simulink model "radiator_model_DOE"  (R2023b)
settings: Solver=FixedStepAuto  StartTime=0.0  StopTime=1200  FixedStep=0.244  RelTol=1e-3
InitFcn:
  | EngHeatRe2EngColnt=2150;
  | ColntFlw=0.2;
  | ColntHeatCp=4200;
  | EngColntMss=5.5;
  | RadColntMss=2.56;
  | RadArea=0.93;
  | AirTemp=13;
  | RadOnFanHgain=9.75;
  | RadH=8;
  | FanOnTemp=91;
  | FanOffTemp=85;
  | TrmstTemp=77.3;
  | InitEngColntOutTemp=55.5;
  | InitRadColntOutTemp=60;
settings Model: Creator=m.sorkhi  LastModifiedBy=m.sorkhi
settings SolverCC: ZeroCrossAlgorithm=Adaptive
settings DebuggingCC: IgnoredZcDiagnostic=none

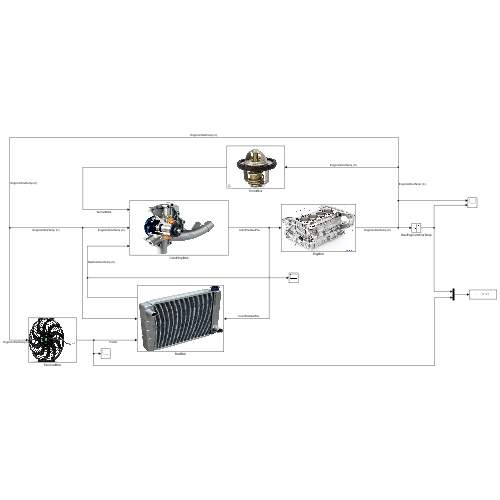
[thumbnail: Simulink's stored preview of the top-level diagram]
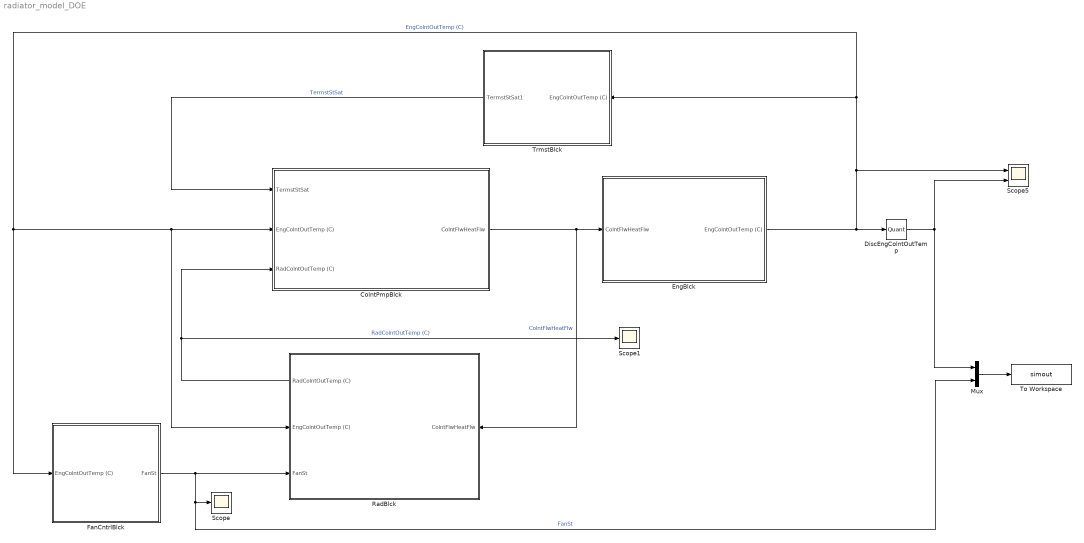
== system radiator_model_DOE ==
  ColntPmpBlck : Subsystem
      mask Display: image('wasserpumpe.jpg');
  DiscEngColntOutTemp : Quantizer  QuantizationInterval=0.75
  EngBlck : Subsystem
      mask Display: image('ICE_engine_block_details.jpg');
  FanCntrlBlck : Subsystem
      mask Display: image('71LbS5WTJxL._AC_UF1000,1000_QL80_.jpg');
  Mux : Mux  Inputs=2
  RadBlck : Subsystem
      settings: PortSchema="{\"entries\":[{\"content\":{\"sides\":[{\"content\":{\"connectorIds\":[\"Out1\",\"In1\",\"In2\"]},\"type\":\"ConnectorPlacement.EquallySpacedRectSide\",\"uuid\":\"5da9f111-79ac-4398-b2ca-ad7113d95e2a\"},{\"content\":{\"connectorIds\":[\"In3\"],\"side\":\"RIGHT\"},\"type\":\"ConnectorPlacement.EquallySpacedRectSide\",\"uuid\":\"beb3da66-0353-45dc-92dd-83812cc99847\"},{\"content\":{\"side\":\"TOP\"},\"type\":\"ConnectorPlacement.EquallySpacedRectSide\",\"uuid\":\"c3de1bb5-6f3a-4f20-91db-640cd95e3994\"}]},\"type\":\"ConnectorPlacement.EquallySpacedConnector\",\"uuid\":\"87d09cf3-4774-453a-a522-35e848abd666\"}],\"packageUris\":[\"http://schema.mathworks.com/mf0/Connector/R2020b\"],\"version\":\"1.0\"}"
      mask Display: image('Automobile_radiator.jpg');
  Scope : Scope
  Scope1 : Scope
  Scope5 : Scope  NumInputPorts=2
  To Workspace : ToWorkspace  VariableName=simout  SaveFormat=Timeseries  SampleTime=-1
  TrmstBlck : Subsystem
      settings: PortSchema="{\"entries\":[{\"content\":{\"sides\":[{\"content\":{\"connectorIds\":[\"Out1\"]},\"type\":\"ConnectorPlacement.EquallySpacedRectSide\",\"uuid\":\"06f11dda-685b-413c-afa7-1258c3976e74\"},{\"content\":{\"connectorIds\":[\"In1\"],\"side\":\"RIGHT\"},\"type\":\"ConnectorPlacement.EquallySpacedRectSide\",\"uuid\":\"2745f48e-69b2-4d48-9193-e2e306ca83ef\"},{\"content\":{\"side\":\"TOP\"},\"type\":\"ConnectorPlacement.EquallySpacedRectSide\",\"uuid\":\"b89a6614-c438-49fa-af5b-58ae8dde8402\"}]},\"type\":\"ConnectorPlacement.EquallySpacedConnector\",\"uuid\":\"ed9858cb-f051-4637-aafc-3b577e7d11cc\"}],\"packageUris\":[\"http://schema.mathworks.com/mf0/Connector/R2020b\"],\"version\":\"1.0\"}"
      mask DialogControl Control1 Prompt: (Add text here)
      mask Display: image('thermostat-a-cooling-system-spare-parts-for-cars-PLFZKVV-min.jpg');
  wires:
  DiscEngColntOutTemp/1 -> Scope5/2, Mux/1
  EngBlck/1(EngColntOutTemp (C)) -> TrmstBlck/1(EngColntOutTemp (C)), ColntPmpBlck/2(EngColntOutTemp (C)), RadBlck/1(EngColntOutTemp (C)), FanCntrlBlck/1(EngColntOutTemp (C)), Scope5/1, DiscEngColntOutTemp/1  "EngColntOutTemp (C)"
  ColntPmpBlck/1(ColntFlwHeatFlw) -> RadBlck/3(ColntFlwHeatFlw), EngBlck/1(ColntFlwHeatFlw)  "ColntFlwHeatFlw"
  RadBlck/1(RadColntOutTemp (C)) -> Scope1/1, ColntPmpBlck/3(RadColntOutTemp (C))  "RadColntOutTemp (C)"
  TrmstBlck/1(TermstStSat1) -> ColntPmpBlck/1(TermstStSat)  "TermstStSat"
  FanCntrlBlck/1(FanSt) -> Mux/2, Scope/1, RadBlck/2(FanSt)  "FanSt"
  Mux/1 -> To Workspace/1

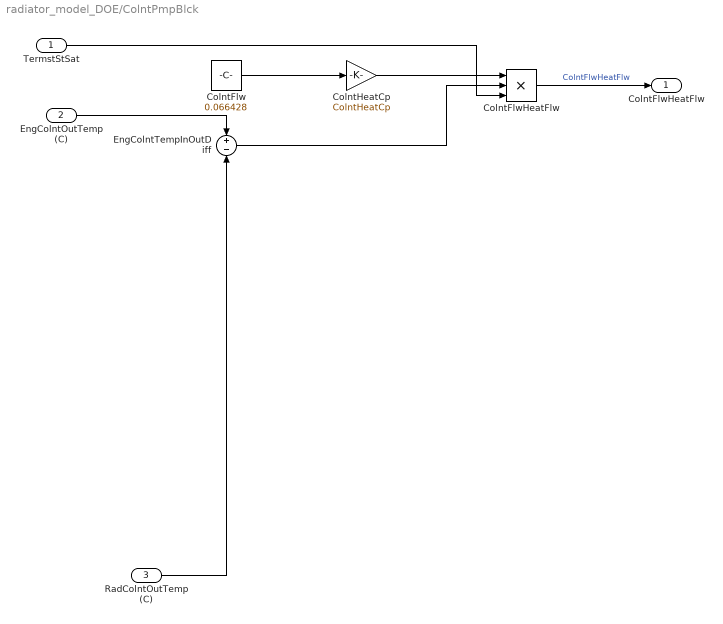
== system radiator_model_DOE/ColntPmpBlck ==
  TermstStSat : Inport
  EngColntOutTemp (C) : Inport  Port=2
  RadColntOutTemp (C) : Inport  Port=3
  ColntFlw : Constant  Value=0.066428
  "ColntFlwHeatFlw " : Product  Inputs=3
  ColntHeatCp : Gain  Gain=ColntHeatCp
  EngColntTempInOutDiff : Sum  Inputs=+-
  ColntFlwHeatFlw : Outport
  wires:
  "ColntFlwHeatFlw "/1 -> ColntFlwHeatFlw/1  "ColntFlwHeatFlw"
  ColntFlw/1 -> ColntHeatCp/1
  EngColntOutTemp (C)/1 -> EngColntTempInOutDiff/1
  ColntHeatCp/1 -> "ColntFlwHeatFlw "/1
  EngColntTempInOutDiff/1 -> "ColntFlwHeatFlw "/2
  TermstStSat/1 -> "ColntFlwHeatFlw "/3
  RadColntOutTemp (C)/1 -> EngColntTempInOutDiff/2

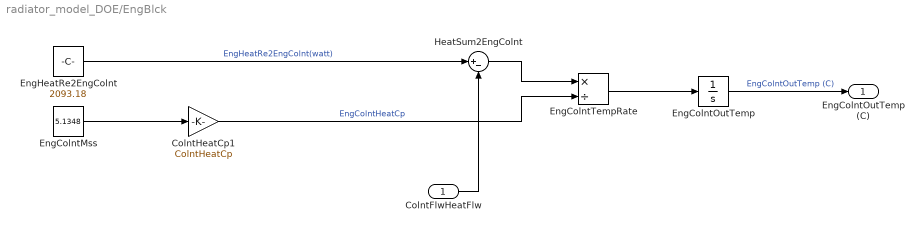
== system radiator_model_DOE/EngBlck ==
  ColntFlwHeatFlw : Inport
  ColntHeatCp1 : Gain  Gain=ColntHeatCp
  EngColntMss : Constant  Value=5.1348
  EngColntOutTemp : Integrator  InitialCondition=InitEngColntOutTemp
  EngColntTempRate : Product  Inputs=*/
  EngHeatRe2EngColnt : Constant  Value=2093.18
  HeatSum2EngColnt : Sum  Inputs=|+-
  EngColntOutTemp (C) : Outport
  wires:
  ColntHeatCp1/1 -> EngColntTempRate/2  "EngColntHeatCp"
  EngColntMss/1 -> ColntHeatCp1/1
  EngColntTempRate/1 -> EngColntOutTemp/1
  ColntFlwHeatFlw/1 -> HeatSum2EngColnt/2
  HeatSum2EngColnt/1 -> EngColntTempRate/1
  EngColntOutTemp/1 -> EngColntOutTemp (C)/1  "EngColntOutTemp (C)"
  EngHeatRe2EngColnt/1 -> HeatSum2EngColnt/1  "EngHeatRe2EngColnt(watt)"

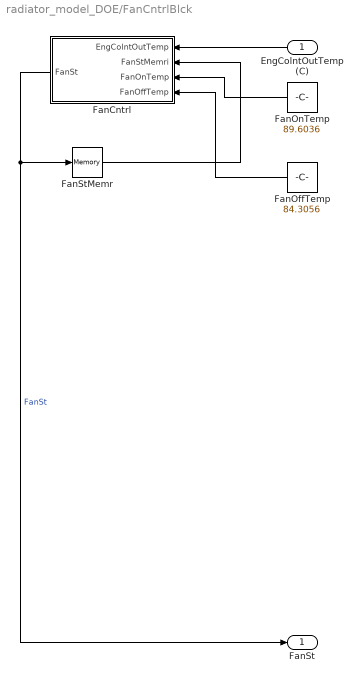
== system radiator_model_DOE/FanCntrlBlck ==
  EngColntOutTemp (C) : Inport
  FanCntrl : MATLAB Function  TreatAsAtomicUnit=on
  FanOffTemp : Constant  Value=84.3056
  FanOnTemp : Constant  Value=89.6036
  "FanStMemr " : Memory
  FanSt : Outport
  wires:
  FanCntrl/1(FanSt) -> FanSt/1, "FanStMemr "/1  "FanSt"
  "FanStMemr "/1 -> FanCntrl/2(FanStMemri)
  EngColntOutTemp (C)/1 -> FanCntrl/1(EngColntOutTemp)
  FanOffTemp/1 -> FanCntrl/4(FanOffTemp)
  FanOnTemp/1 -> FanCntrl/3(FanOnTemp)

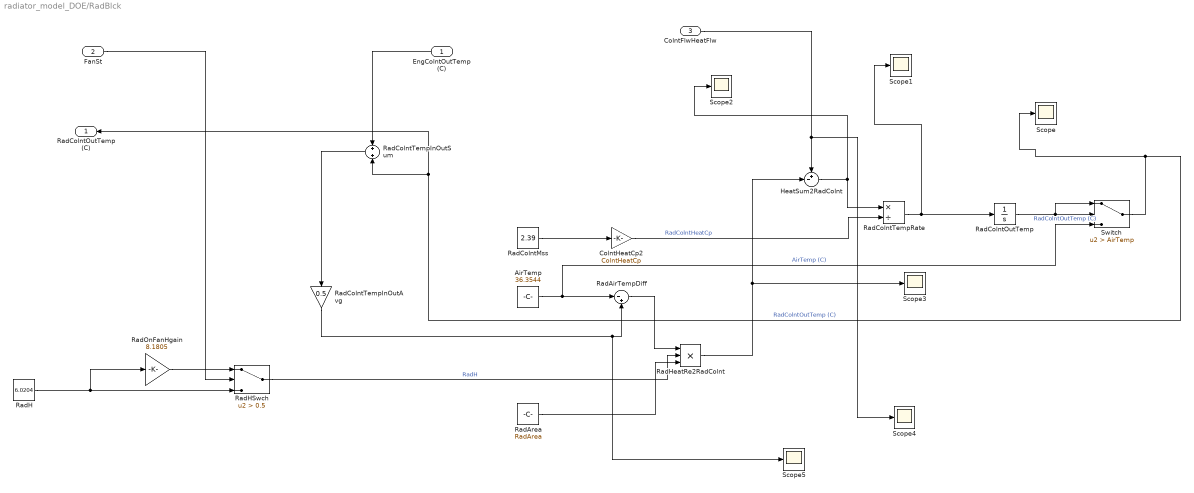
== system radiator_model_DOE/RadBlck ==
  EngColntOutTemp (C) : Inport
  FanSt : Inport  Port=2
  ColntFlwHeatFlw : Inport  Port=3
  AirTemp : Constant  Value=36.3544
  ColntHeatCp2 : Gain  Gain=ColntHeatCp
  HeatSum2RadColnt : Sum  Inputs=+-|
  RadAirTempDiff : Sum  Inputs=|-+
  RadArea : Constant  Value=RadArea
  RadColntMss : Constant  Value=2.39
  RadColntOutTemp : Integrator  InitialCondition=InitRadColntOutTemp
  RadColntTempInOutAvg : Gain  Gain=0.5
  RadColntTempInOutSum : Sum  Inputs=+|+
  RadColntTempRate : Product  Inputs=*/
  RadH : Constant  Value=6.0204
  RadHSwch : Switch  Criteria=u2 > Threshold  Threshold=0.5  SaturateOnIntegerOverflow=off  InputSameDT=off
  RadHeatRe2RadColnt : Product  Inputs=3
  RadOnFanHgain : Gain  Gain=8.1805
  Scope{,1..5} (6 alike) : Scope
  Switch : Switch  Criteria=u2 > Threshold  Threshold=AirTemp  SaturateOnIntegerOverflow=off  InputSameDT=off
  RadColntOutTemp (C) : Outport
  wires:
  RadColntTempInOutAvg/1 -> Scope5/1, RadAirTempDiff/2
  AirTemp/1 -> Switch/3, RadAirTempDiff/1  "AirTemp (C)"
  RadAirTempDiff/1 -> RadHeatRe2RadColnt/1
  RadColntMss/1 -> ColntHeatCp2/1
  Switch/1 -> Scope/1, RadColntOutTemp (C)/1, RadColntTempInOutSum/2  "RadColntOutTemp (C)"
  RadHeatRe2RadColnt/1 -> HeatSum2RadColnt/2, Scope3/1
  HeatSum2RadColnt/1 -> RadColntTempRate/1, Scope2/1
  RadHSwch/1 -> RadHeatRe2RadColnt/2  "RadH"
  RadColntTempRate/1 -> Scope1/1, RadColntOutTemp/1
  RadArea/1 -> RadHeatRe2RadColnt/3
  RadColntTempInOutSum/1 -> RadColntTempInOutAvg/1
  ColntHeatCp2/1 -> RadColntTempRate/2  "RadColntHeatCp"
  RadH/1 -> RadOnFanHgain/1, RadHSwch/3
  FanSt/1 -> RadHSwch/2
  EngColntOutTemp (C)/1 -> RadColntTempInOutSum/1
  ColntFlwHeatFlw/1 -> Scope4/1, HeatSum2RadColnt/1
  RadColntOutTemp/1 -> Switch/2, Switch/1  "RadColntOutTemp (C)"
  RadOnFanHgain/1 -> RadHSwch/1

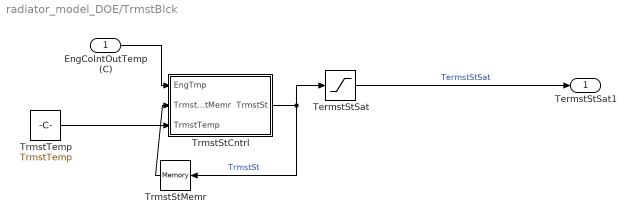
== system radiator_model_DOE/TrmstBlck ==
  EngColntOutTemp (C) : Inport
  TermstStSat : Saturate  UpperLimit=1  LowerLimit=0
  "TrmstStCntrl " : MATLAB Function  TreatAsAtomicUnit=on
  "TrmstStMemr " : Memory
  TrmstTemp : Constant  Value=TrmstTemp
  TermstStSat1 : Outport
  wires:
  "TrmstStMemr "/1 -> "TrmstStCntrl "/2(TrmstStMemr)
  "TrmstStCntrl "/1(TrmstSt) -> "TrmstStMemr "/1, TermstStSat/1  "TrmstSt"
  TermstStSat/1 -> TermstStSat1/1  "TermstStSat"
  EngColntOutTemp (C)/1 -> "TrmstStCntrl "/1(EngTmp)
  TrmstTemp/1 -> "TrmstStCntrl "/3(TrmstTemp)

== matlab function radiator_model_DOE/TrmstBlck/TrmstStCntrl  ==
  data: EngTmp input; TrmstSt output; TrmstStMemr input; TrmstTemp input
function TrmstSt= fcn(EngTmp,TrmstStMemr,TrmstTemp)
    if EngTmp>=TrmstTemp
        TrmstSt=0.1*EngTmp-(TrmstTemp-5)/10;
    elseif EngTmp<=(TrmstTemp-5)
        TrmstSt=0;
    elseif EngTmp < TrmstTemp && EngTmp>(TrmstTemp-5) && TrmstStMemr>0
        TrmstSt=0.1*EngTmp-(TrmstTemp-5)/10;
    else 
        TrmstSt=0;
    end
end

== matlab function radiator_model_DOE/FanCntrlBlck/FanCntrl ==
  data: EngColntOutTemp input; FanSt output; FanStMemri input; FanOnTemp input; FanOffTemp input
function FanSt = fcn(EngColntOutTemp,FanStMemri,FanOnTemp,FanOffTemp)
    if EngColntOutTemp>=FanOnTemp
        FanSt=1;
    elseif EngColntOutTemp < FanOffTemp
        FanSt=0;
    elseif EngColntOutTemp < FanOnTemp && EngColntOutTemp>= FanOffTemp && FanStMemri == 1
        FanSt=1;
    else 
        FanSt=0;
    end
end
